simulink model "lab02Daqtest"  (R2016b)
settings: Solver=ode3  StartTime=0.0  StopTime=inf  FixedStep=Ts  RelTol=1e-3  EnableMultiTasking=on
libraries: Rayannik x7
settings Model: SimulationMode=external  ExtModeTrigDuration=1000001  Creator=user  LastModifiedBy=Alireza7
settings DataIOCC: LimitDataPoints=on  SaveFormat=Array
settings DebuggingCC: SolverPrmCheckMsg=warning  SFUnexpectedBacktrackingDiag=warning  SFNoUnconditionalDefaultTransitionDiag=warning  SFExecutionAtInitializationDiag=none
settings ModelReferenceCC: PropagateSignalLabelsOutOfModel=off
settings RTWCC: SystemTargetFile=sldrt.tlc  TemplateMakefile=sldrt.tmf  Description=Simulink Desktop Real-Time  RTWCompilerOptimization=on
settings CodeAppCC: MaxIdLength=95
settings SimulinkDesktopRealTimeCC: TargetPreCompLibLocation=C:\Program Files\MATLAB\R2016b\toolbox\sldrt\lib\win64  TargetLangStandard=C89/C90 (ANSI)  SupportVariableSizeSignals=off
settings ConfigComp: CovMetricSettings=dw  CovHtmlReporting=on  CovSaveCumulativeToWorkspaceVar=on  CovSaveSingleToWorkspaceVar=on  CovExternalEMLEnable=off  CovSFcnEnable=off

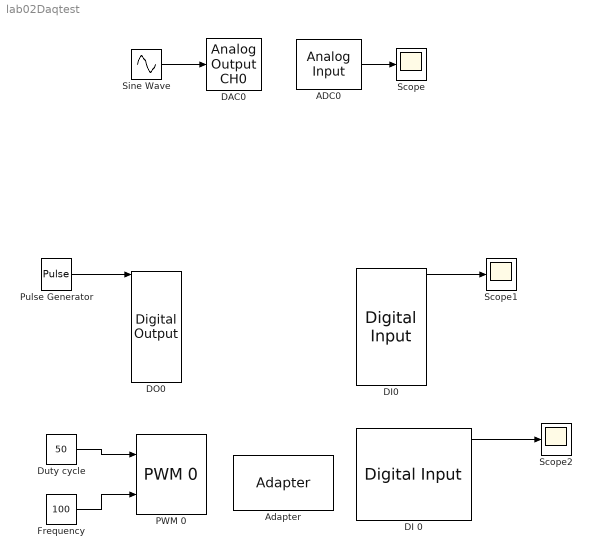
== system lab02Daqtest ==
  ADC0 : Rayannik/Analog Input  Priority=2  CH=0  vr=2.5  ou=Analog  inrr=-10 ~ +10
  Adapter : Rayannik/Adapter  SystemSampleTime=-1
      link override Packet Input1: SampleTime=Ts  MaxMissedTicks=1000000  ShowMissedTicks=off  YieldWhenWaiting=off  DrvName=Standard_Devices/Serial_Port  DrvAddress=3  DrvOptions=[9600 8 0 0 0 0 0 0]  PacketSize=33  DataTypes='33*uint8'  ShowReady=off  ShowError=off  PacketID=1  ByteOrder=1  ShowTimestamp=off
      link override Packet Output1: SampleTime=Ts  MaxMissedTicks=10000000  ShowMissedTicks=off  YieldWhenWaiting=off  DrvName=Standard_Devices/Serial_Port  DrvAddress=3  DrvOptions=[9600 8 0 0 0 0 0 0]  PacketSize=31  DataTypes='31*uint8'  ShowReady=off  ShowError=off  PacketID=1  ByteOrder=1  InitialValue=[]  FinalValue=[]
  DAC0 : Rayannik/Analog Output CH0  Priority=2  rfo=2.5  inpm=Analog  inr=-10 ~ +10
  DI 0 : Rayannik/Digital Input  Priority=2
  DI0 : Rayannik/Digital Input  Priority=2
  DO0 : Rayannik/Digital Output  Priority=2
  Duty cycle : Constant  Value=50
  Frequency : Constant  Value=100
  PWM 0 : Rayannik/PWM 0  Priority=2  md=Constant Frequency Mode
  Pulse Generator : DiscretePulseGenerator  PulseType=Time based  Amplitude=5  PulseWidth=50
  Scope : Scope
  Scope1 : Scope
  Scope2 : Scope
  Sine Wave : Sin  Amplitude=2  SampleTime=0
  wires:
  ADC0/1 -> Scope/1
  Sine Wave/1 -> DAC0/1
  DI0/1 -> Scope1/1
  Pulse Generator/1 -> DO0/1
  DI 0/1 -> Scope2/1
  Frequency/1 -> PWM 0/2
  Duty cycle/1 -> PWM 0/1
